simulink model "sla_VHT_ref"  (R2015b)
settings: Solver=FixedStepDiscrete  SolverMode=SingleTasking  StartTime=0.0  StopTime=320*240*100  RelTol=1e-3
PreLoadFcn:
  | H = fspecial('unsharp')
undefined symbols (not defined in the file or in its folder): gray
libraries: visionsinks x3, visionconversions x2, visionfilter x1, dspvision x1
settings Model: Creator=yutengz  LastModifiedBy=amatsumo
settings DataIOCC: SaveFormat=Array
settings OptimizationCC: BlockReduction=off  BooleanDataType=off
settings DebuggingCC: SaveWithParameterizedLinksMsg=none  UnderspecifiedInitializationDetection=Classic  MergeDetectMultiDrivingBlocksExec=none  SignalResolutionControl=TryResolveAllWithWarning
settings HardwareCC: ProdBitPerPointer=32  ProdLargestAtomicFloat=None  ProdIntDivRoundTo=Undefined  ProdEndianess=Unspecified  ProdWordSize=32  ProdHWDeviceType=32-bit Generic  TargetUnknown=on
settings GRTTargetCC: GeneratePreprocessorConditionals=Disable all
settings ConfigComp: CovModelRefEnable=Off  CovSFcnEnable=off

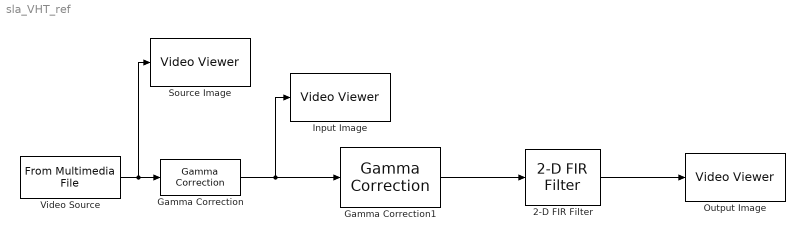
== system sla_VHT_ref ==
  2-D FIR Filter : visionfilter/2-D FIR Filter  separable=off  filtSrc=Specify via dialog  filterMtrx=H  verticalFilter=[4 0]  horizontalFilter=[4 0]  outSize=Same as input port I  padType=Constant  padSrc=Specify via dialog  padVal=0  method=Convolution  firstCoeffMode=Binary point scaling  firstCoeffWordLength=8  firstCoeffFracLength=4  firstCoeffSignedness=Signed  firstCoeffDataTypeStr=fixdt(1,8,4)  firstCoeffLastDataTypeStr=fixdt(1,8,4)  firstCoeffMin=[]  firstCoeffMax=[]  outputSignedness=Auto  outputMin=[]  outputMax=[]  accumDataTypeStr=Inherit: Same as product output  accumLastDataTypeStr=Inherit: Same as product output  prodOutputMode=Binary point scaling  prodOutputWordLength=32  prodOutputFracLength=10  prodOutputDataTypeStr=fixdt([],32,10)  prodOutputLastDataTypeStr=fixdt([],32,10)  roundingMode=Floor  overflowMode=on
  Gamma Correction : visionconversions/Gamma Correction  operation=De-gamma  gamma=2.2  linearSegment=on  breakPoint=0.018
  Gamma Correction1 : visionconversions/Gamma Correction  operation=Gamma  gamma=2.2  linearSegment=on  breakPoint=0.018
  Input Image : visionsinks/Video Viewer  inputType=Obsolete7b  imagePorts=One multidimensional signal  useColorMap=off  colormapValue=gray(256)  specRange=off  minInputVal=0  maxInputVal=255  FigPos=[366 381 334 275]  AxisZoom=on  trueSizedOnce=off  OpenAtMdlStart=on  DefaultConfigurationName=vipscopes.VideoViewerScopeCfg
  Output Image : visionsinks/Video Viewer  inputType=Obsolete7b  imagePorts=One multidimensional signal  useColorMap=off  colormapValue=gray(256)  specRange=off  minInputVal=0  maxInputVal=255  FigPos=[710 382 334 275]  AxisZoom=on  trueSizedOnce=off  OpenAtMdlStart=on  DefaultConfigurationName=vipscopes.VideoViewerScopeCfg
  Source Image : visionsinks/Video Viewer  inputType=Obsolete7b  imagePorts=One multidimensional signal  useColorMap=off  colormapValue=gray(256)  specRange=off  minInputVal=0  maxInputVal=255  FigPos=[21 379 334 275]  AxisZoom=on  trueSizedOnce=off  OpenAtMdlStart=on  DefaultConfigurationName=vipscopes.VideoViewerScopeCfg
  Video Source : dspvision/From Multimedia File  inputFilename=rhinos.avi  loop=on  numPlays=inf  outputStreams=Video only  videoDataType=uint8  audioDataType=int16  inheritSampleTime=off  userDefinedSampleTime=402*324  noAudioOutput=off  isIntensityVideo=off  fourcc=Intensity  colorVideoFormat=One multidimensional signal  outputEOF=off  dataOrg=Column-major  audioFrameSize=1024  computeAudioFrameSize=off  outSamplingMode=Sample based
  wires:
  Video Source/1 -> Source Image/1, Gamma Correction/1
  2-D FIR Filter/1 -> Output Image/1
  Gamma Correction/1 -> Gamma Correction1/1, Input Image/1
  Gamma Correction1/1 -> 2-D FIR Filter/1
